simulink model "commander"  (R2021a)
settings: Solver=FixedStepAuto  StartTime=0.0  StopTime=5  FixedStep=0.02  RelTol=1e-3
(part 1 of 2)
settings Model: DataDictionary=px4_dict.sldd  Creator=DELL  LastModifiedBy=DELL
settings OptimizationCC: DefaultParameterBehavior=Inlined  EnhancedBackFolding=on  PassReuseOutputArgsAs=Individual arguments  ZeroExternalMemoryAtStartup=off  ZeroInternalMemoryAtStartup=off  OptimizeBlockOrder=speed  DifferentSizesBufferReuse=on  OptimizationCustomize=off  EfficientTunableParamExpr=on
settings DebuggingCC: ParameterPrecisionLossMsg=none  ParameterTunabilityLossMsg=error  UnitsInconsistencyMsg=none
settings SFSimCC: MATLABDynamicMemAlloc=off
settings RTWCC: SystemTargetFile=ert.tlc  TemplateMakefile=ert_default_tmf
settings CodeAppCC: ForceParamTrailComments=on  IgnoreCustomStorageClasses=off  OperatorAnnotations=on  SimulinkDataObjDesc=on  SFDataObjDesc=on  InsertBlockDesc=on
settings ERTTargetCC: TargetLangStandard=C99 (ISO)  GenerateSampleERTMain=on  InlinedParameterPlacement=NonHierarchical  ERTCustomFileTemplate=example_file_process.tlc

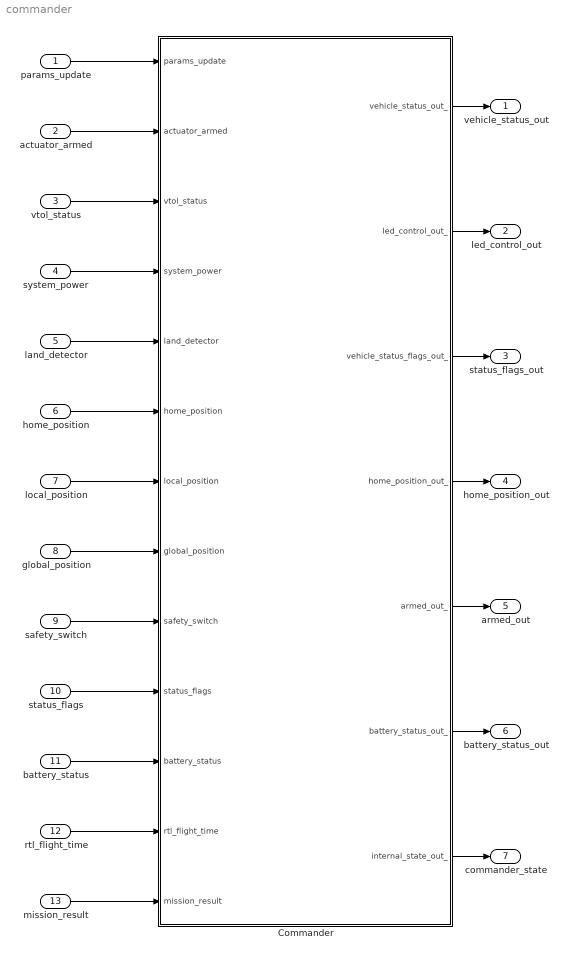
== system commander ==
  params_update : Inport  OutDataTypeStr=Bus: px4_parameter_update  BusOutputAsStruct=on
  actuator_armed : Inport  Port=2  OutDataTypeStr=Bus: px4_actuator_armed  BusOutputAsStruct=on
  vtol_status : Inport  Port=3  OutDataTypeStr=Bus: px4_vtol_vehicle_status  BusOutputAsStruct=on
  system_power : Inport  Port=4  OutDataTypeStr=Bus: px4_system_power  BusOutputAsStruct=on
  land_detector : Inport  Port=5  OutDataTypeStr=Bus: px4_vehicle_land_detected  BusOutputAsStruct=on
  home_position : Inport  Port=6  OutDataTypeStr=Bus: px4_home_position  BusOutputAsStruct=on
  local_position : Inport  Port=7  OutDataTypeStr=Bus: px4_vehicle_local_position  BusOutputAsStruct=on
  global_position : Inport  Port=8  OutDataTypeStr=Bus: px4_vehicle_global_position  BusOutputAsStruct=on
  safety_switch : Inport  Port=9  OutDataTypeStr=Bus: px4_safety  BusOutputAsStruct=on
  status_flags : Inport  Port=10  OutDataTypeStr=Bus: px4_vehicle_status_flags  BusOutputAsStruct=on
  battery_status : Inport  Port=11  OutDataTypeStr=Bus: px4_battery_status  BusOutputAsStruct=on
  rtl_flight_time : Inport  Port=12  OutDataTypeStr=Bus: px4_rtl_flight_time  BusOutputAsStruct=on
  mission_result : Inport  Port=13  OutDataTypeStr=Bus: px4_mission_result  BusOutputAsStruct=on
  Commander : Stateflow chart  TreatAsAtomicUnit=on
  vehicle_status_out : Outport  OutDataTypeStr=Bus: px4_vehicle_status  BusOutputAsStruct=on
  led_control_out : Outport  Port=2  OutDataTypeStr=Bus: px4_led_control  BusOutputAsStruct=on
  status_flags_out : Outport  Port=3  OutDataTypeStr=Bus: px4_vehicle_status_flags  BusOutputAsStruct=on
  home_position_out : Outport  Port=4  OutDataTypeStr=Bus: px4_home_position  BusOutputAsStruct=on
  armed_out : Outport  Port=5  OutDataTypeStr=Bus: px4_actuator_armed  BusOutputAsStruct=on
  battery_status_out : Outport  Port=6  OutDataTypeStr=Bus: px4_battery_status  BusOutputAsStruct=on
  commander_state : Outport  Port=7  OutDataTypeStr=Bus: px4_commander_state  BusOutputAsStruct=on
  wires:
  mission_result/1 -> Commander/13(mission_result)
  rtl_flight_time/1 -> Commander/12(rtl_flight_time)
  battery_status/1 -> Commander/11(battery_status)
  Commander/7(internal_state_out_) -> commander_state/1
  actuator_armed/1 -> Commander/2(actuator_armed)
  params_update/1 -> Commander/1(params_update)
  Commander/6(battery_status_out_) -> battery_status_out/1
  Commander/5(armed_out_) -> armed_out/1
  safety_switch/1 -> Commander/9(safety_switch)
  status_flags/1 -> Commander/10(status_flags)
  global_position/1 -> Commander/8(global_position)
  local_position/1 -> Commander/7(local_position)
  Commander/3(vehicle_status_flags_out_) -> status_flags_out/1
  Commander/4(home_position_out_) -> home_position_out/1
  land_detector/1 -> Commander/5(land_detector)
  home_position/1 -> Commander/6(home_position)
  vtol_status/1 -> Commander/3(vtol_status)
  system_power/1 -> Commander/4(system_power)
  Commander/1(vehicle_status_out_) -> vehicle_status_out/1
  Commander/2(led_control_out_) -> led_control_out/1
